simulink model "gama"  (R2020a)
settings: Solver=ode45  StartTime=0.0  StopTime=10.0  RelTol=1e-3
values from neighbouring files (symbols this model uses):
  g = 9.807    [parameters.m]
  gam_0 = pi/2    (= 1.57079632679)    [parameters.m]
  gam_in = 0.1    [parameters.m]
  h_0 = 0    [parameters.m]
  m_dot = 132    [parameters.m]
  m_zfw = m_pay+m_dry    (= 6360.7)    [parameters.m]
  R_E = 6371e3    (= 6371000)    [parameters.m]
  t_turn = 30    [parameters.m]
  v_0 = 0.01    [parameters.m]
  x_0 = 0    [parameters.m]
libraries: simulink x2
settings Model: Creator=benyo  LastModifiedBy=benyo

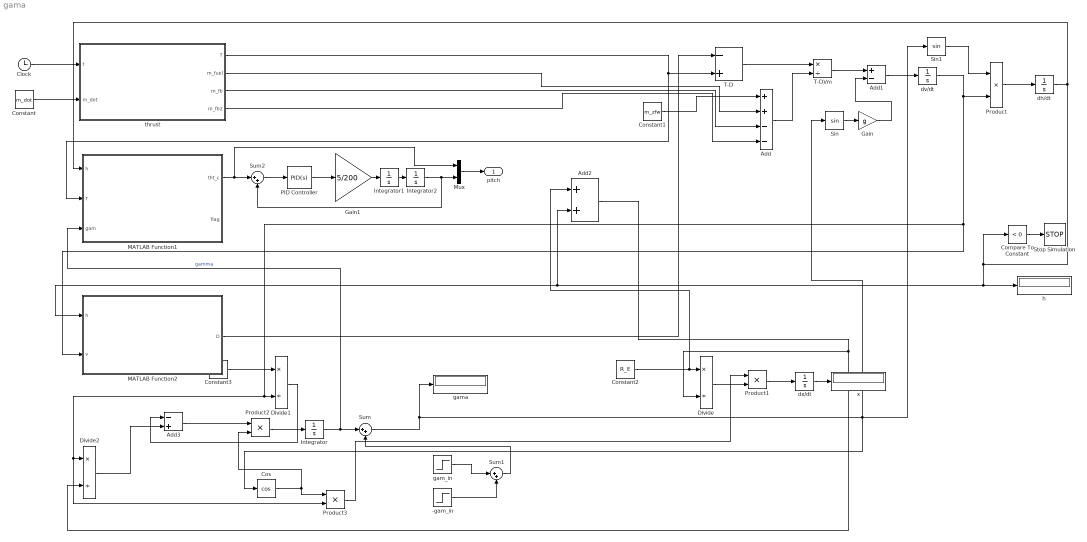
== system gama ==
  -gam_in : Step  Time=t_turn+1  Before=-gam_in  After=-gam_in  SampleTime=0
  Add : Sum  Inputs=++--
  Add1 : Sum  Inputs=+-
  Add2 : Sum
  Add3 : Sum  Inputs=-+
  Clock : Clock
  Compare To Constant : simulink/Logic and Bit Operations/Compare To Constant  relop=<  const=0  OutDataTypeStr=boolean
  Constant : Constant  Value=m_dot
  Constant1 : Constant  Value=m_zfw
  Constant2 : Constant  Value=R_E
  Constant3 : Constant  Value=g
  Cos : Trigonometry  Operator=cos
  Divide : Product  Inputs=*/
  Divide1 : Product  Inputs=*/
  Divide2 : Product  Inputs=*/
  Gain : Gain  Gain=g
  Gain1 : Gain  Gain=5/200
  Integrator : Integrator  InitialCondition=gam_0
  Integrator1 : Integrator
  Integrator2 : Integrator  InitialCondition=pi/2
  MATLAB Function1 : MATLAB Function  TreatAsAtomicUnit=on
  MATLAB Function2 : MATLAB Function  TreatAsAtomicUnit=on
  Mux : Mux  Inputs=2
  PID Controller : simulink/Continuous/PID Controller  Controller=PID  Form=Parallel  TimeDomain=Continuous-time  UseExternalTs=off  SampleTime=-1  IntegratorMethod=Forward Euler  FilterMethod=Forward Euler  ControllerParametersSource=internal  P=0  I=0  D=200/5  UseFilter=on  N=100  TunerSelectOption=Transfer Function Based (PID Tuner App)  InitialConditionSource=internal  InitialConditionForIntegrator=0  InitialConditionForFilter=0  DifferentiatorICPrevScaledInput=0  ExternalReset=none  TrackingMode=off  Kt=1  LimitOutput=off  UpperSaturationLimit=inf  LowerSaturationLimit=-inf  LinearizeAsGain=on  AntiWindupMode=none  Kb=1  POutMin=[]  POutMax=[]  IOutMin=[]  IOutMax=[]  DOutMin=[]  DOutMax=[]  NOutMin=[]  NOutMax=[]  SumOutMin=[]  SumOutMax=[]  SaturationOutMin=[]  SaturationOutMax=[]  PParamMin=[]  PParamMax=[]  IParamMin=[]  IParamMax=[]  DParamMin=[]  DParamMax=[]  NParamMin=[]  NParamMax=[]  KbParamMin=[]  KbParamMax=[]  KtParamMin=[]  KtParamMax=[]  KbOutMin=[]  KbOutMax=[]  KtOutMin=[]  KtOutMax=[]  IntegratorOutMin=[]  IntegratorOutMax=[]  FilterOutMin=[]  FilterOutMax=[]  SumI1OutMin=[]  SumI1OutMax=[]  SumI2OutMin=[]  SumI2OutMax=[]  SumI3OutMin=[]  SumI3OutMax=[]  SumI4OutMin=[]  SumI4OutMax=[]  SumDOutMin=[]  SumDOutMax=[]  DifferentiatorOutMin=[]  DifferentiatorOutMax=[]  FilterDiffOutCoefMin=[]  FilterDiffOutCoefMax=[]  ReciprocalOutMin=[]  ReciprocalOutMax=[]  SumDenOutMin=[]  SumDenOutMax=[]  SumNumOutMin=[]  SumNumOutMax=[]  DivideOutMin=[]  DivideOutMax=[]  UdiffTsProdOutMin=[]  UdiffTsProdOutMax=[]  NTsProdOutMin=[]  NTsProdOutMax=[]  UintegralTsProdOutMin=[]  UintegralTsProdOutMax=[]  UngainTsProdOutMin=[]  UngainTsProdOutMax=[]  IntegratorContinuousStateAttributes=''  IntegratorStateMustResolveToSignalObject=off  IntegratorRTWStateStorageClass=Auto  FilterContinuousStateAttributes=''  FilterStateMustResolveToSignalObject=off  FilterRTWStateStorageClass=Auto  ParallelPVariant=InternalParameters  IdealPVariant=Disabled  IVariant=InternalParameters  DVariant=InternalParameters  IntegratorVariant=Continuous  SatVariant=Disabled  AWVariant=Passthrough  PCopyVariant=Disabled  TRVariant=Disabled  FdbkBlocksVariant=Forward  IdealPFdbkVariant=Disabled  SatFdbkVariant=Disabled  DerivativeFilterVariant=ContFilter  NVariant=InternalParameters  NCopyVariant=Disabled  FilterICVariant=InternalICsFilter  IntegratorICVariant=InternalICs  ExternalResetVariant=Disabled  TRSumVariant=Passthrough  SumFdbkVariant=Disabled  SumVariant=Sum_PID  TsampFilterVariant=InternalTs  TsampNgainVariant=Passthrough  TsampIntegralVariant=Passthrough
  Product{,1..3} (4 alike) : Product
  Sin : Trigonometry
  Sin1 : Trigonometry
  Stop Simulation : Stop
  Sum : Sum  Inputs=|++
  Sum1 : Sum  Inputs=|++
  Sum2 : Sum  Inputs=|++
  T-D : Sum  Inputs=-+
  T-D)/m : Product  Inputs=*/
  dh/dt : Integrator  InitialCondition=h_0
  dv/dt : Integrator  InitialCondition=v_0
  dx/dt : Integrator  InitialCondition=x_0
  gam_in : Step  Time=t_turn  Before=gam_in  After=0  SampleTime=0
  gama : Display
  h : Display
  thrust : MATLAB Function  TreatAsAtomicUnit=on
  x : Display
  pitch : Outport
  wires:
  Clock/1 -> thrust/1(t)
  Constant/1 -> thrust/2(m_dot)
  thrust/1(T) -> MATLAB Function1/2(T), T-D/2
  Constant1/1 -> Add/1
  thrust/2(m_fuel) -> Add/2
  thrust/3(m_fb) -> Add/3
  thrust/4(m_fb2) -> Add/4
  T-D/1 -> T-D)/m/1
  Add/1 -> T-D)/m/2
  T-D)/m/1 -> Add1/1
  Sin/1 -> Gain/1
  Add1/1 -> dv/dt/1
  dv/dt/1 -> Product3/2, Divide2/1, Divide1/2, MATLAB Function2/2(v), Product/2
  Product/1 -> dh/dt/1
  dh/dt/1 -> h/1, MATLAB Function2/1(h), Add2/2, Compare To Constant/1, MATLAB Function1/1(h)
  Compare To Constant/1 -> Stop Simulation/1
  MATLAB Function2/1(D) -> T-D/1
  Constant2/1 -> Add2/1, Divide/1
  Add2/1 -> Divide2/2, Divide/2
  Divide/1 -> Product1/2
  Product1/1 -> dx/dt/1
  Constant3/1 -> Divide1/1
  Gain/1 -> Add1/2
  Divide2/1 -> Add3/2
  Divide1/1 -> Add3/1
  Add3/1 -> Product2/1
  Product2/1 -> Integrator/1
  Integrator/1 -> MATLAB Function1/3(gam), Sum/1  "gamma"
  Sum/1 -> Sin1/1, Cos/1, Sin/1, gama/1
  Cos/1 -> Product3/1, Product2/2
  Product3/1 -> Product1/1
  Sin1/1 -> Product/1
  gam_in/1 -> Sum1/1
  -gam_in/1 -> Sum1/2
  Sum1/1 -> Sum/2
  MATLAB Function1/1(tht_c) -> Mux/1, Sum2/1
  PID Controller/1 -> Gain1/1
  Sum2/1 -> PID Controller/1
  Gain1/1 -> Integrator1/1
  Integrator1/1 -> Integrator2/1
  Integrator2/1 -> Mux/2, Sum2/2
  Mux/1 -> pitch/1
  dx/dt/1 -> x/1

== matlab function gama/MATLAB Function1 ==
  data: h input; tht_c output; T input; gam input; flag output
function [tht_c, flag] = fcn(h, T, gam)

persistent f
if isempty(f)
    f=0;
end

if T<=0
    t_c =gam+pi;
    if t_c>pi
        t_c=pi;
    end
    f=1;
elseif T<=0 && h<1000
    t_c=pi/2;
else
    t_c=gam;
end
flag=f;
tht_c=t_c;

== matlab function gama/thrust ==
  data: t input; T output; m_fuel output; m_fb output; m_fb2 output; m_dot input
function [T, m_fuel, m_fb, m_fb2] = fcn(t, m_dot)
persistent mfb
persistent mfb2
if isempty(mfb)
mfb=0;
end
if isempty(mfb2)
mfb2=0;
end
mfuel=21491.26;

if mfb <= 0.65*mfuel
    THR=346961.2;
    mfb=t*m_dot;
else
    THR=0;
end

if(125<t) && (t<295)
    THR=-110000;
    mfb2=(t-125)*(m_dot/3);
end

T=THR;
m_fb=mfb;
m_fb2=mfb2;
m_fuel=mfuel;
y = u;

== matlab function gama/MATLAB Function2 ==
  data: h input; D output; v input
function D = fcn(h,v)

Cd=0.075;
Dia=1.5;
A=pi*Dia^2/4;

%density model
if h<=11000
    T=15.04-0.00649*h;
    p=101.29*((T+273.1)/288.08)^5.258;
elseif (11000<h) && (h<=25000)
    T=-56.46;
    p=22.65*exp(1.73-0.000157*h);
else
    T=-131.21+ 0.00299*h;
    p=2.488*((T+273.1)/216.6)^-11.388;
end

rho=p/(0.2869*(T+273.1));

%DRAG FORCE D

Drag=0.5*rho*v^2*A*Cd;

D = Drag;
